simulink model "P3_sim"  (R2020b)
settings: Solver=VariableStepAuto  StartTime=0.0  StopTime=25  FixedStep=0.1  RelTol=1e-3
model workspace (MAT data in the model file):
  eslasticidade = 0
  teste = 0
libraries: simulink x1
settings Model: Creator=Tiago  LastModifiedBy=Utilizador
settings SolverCC: ZeroCrossAlgorithm=Adaptive
settings DataIOCC: SaveState=on
settings DebuggingCC: IgnoredZcDiagnostic=none

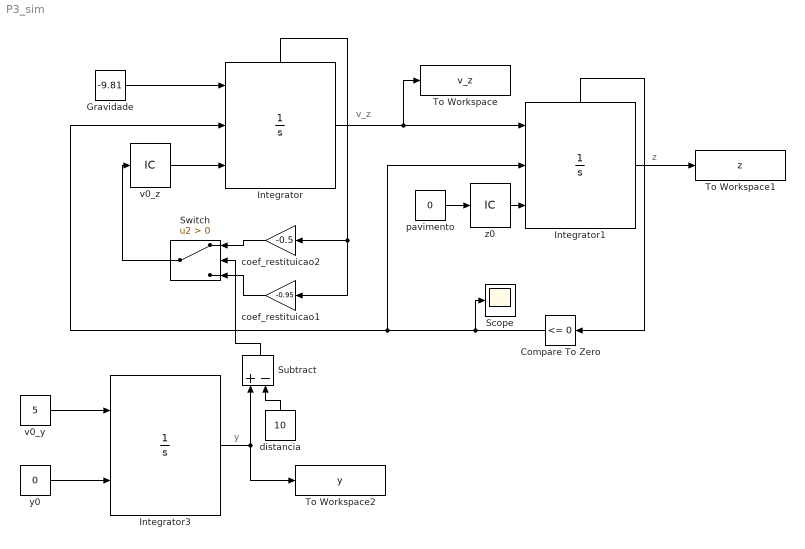
== system P3_sim ==
  note: z
  note: v_z
  note: y
  Compare To Zero : simulink/Logic and Bit Operations/Compare To Zero  relop=<=  OutDataTypeStr=boolean
  Gravidade : Constant  Value=-9.81
  Integrator : Integrator  ExternalReset=rising  InitialConditionSource=external  ShowStatePort=on  ContinuousStateAttributes='Velocidade'
  Integrator1 : Integrator  ExternalReset=rising  InitialConditionSource=external  ShowStatePort=on
  Integrator3 : Integrator  InitialConditionSource=external
  Scope : Scope
  Subtract : Sum  Inputs=+-
  Switch : Switch  Criteria=u2 > Threshold
  To Workspace : ToWorkspace  VariableName=v_z  SaveFormat=Timeseries  SampleTime=-1
  To Workspace1 : ToWorkspace  VariableName=z  SaveFormat=Timeseries  SampleTime=-1
  To Workspace2 : ToWorkspace  VariableName=y  SaveFormat=Timeseries  SampleTime=-1
  coef_restituicao1 : Gain  Tag=teste  Gain=-0.95
  coef_restituicao2 : Gain  Tag=teste  Gain=-0.5
  distancia : Constant  Value=10
  pavimento : Constant  Value=0
  v0_y : Constant  Value=5
  v0_z : InitialCondition  Value=0
  y0 : Constant  Value=0
  z0 : InitialCondition  Value=10
  wires:
  Gravidade/1 -> Integrator/1
  v0_z/1 -> Integrator/3
  Integrator/State -> coef_restituicao1/1, coef_restituicao2/1
  Integrator/1 -> To Workspace/1, Integrator1/1
  z0/1 -> Integrator1/3
  pavimento/1 -> z0/1
  Integrator1/State -> Compare To Zero/1
  Compare To Zero/1 -> Integrator/2, Integrator1/2, Scope/1
  Integrator1/1 -> To Workspace1/1
  v0_y/1 -> Integrator3/1
  Integrator3/1 -> To Workspace2/1, Subtract/1
  coef_restituicao1/1 -> Switch/3
  Switch/1 -> v0_z/1
  y0/1 -> Integrator3/2
  coef_restituicao2/1 -> Switch/1
  distancia/1 -> Subtract/2
  Subtract/1 -> Switch/2
